simulink model "level1_challenge2a"  (R2023b)
settings: Solver=VariableStepAuto  StartTime=0.0  StopTime=600  RelTol=1e-3
settings Model: Creator=evreng  LastModifiedBy=evreng

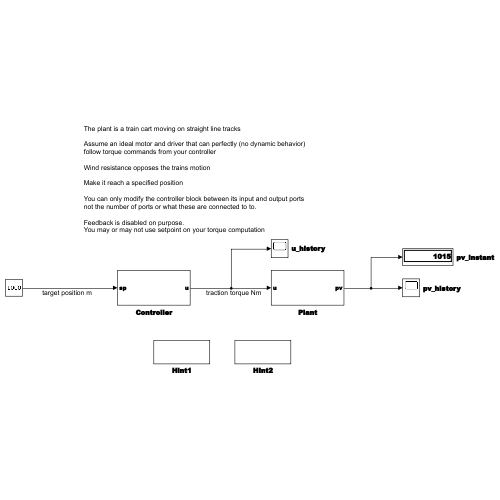
[thumbnail: Simulink's stored preview of the top-level diagram]
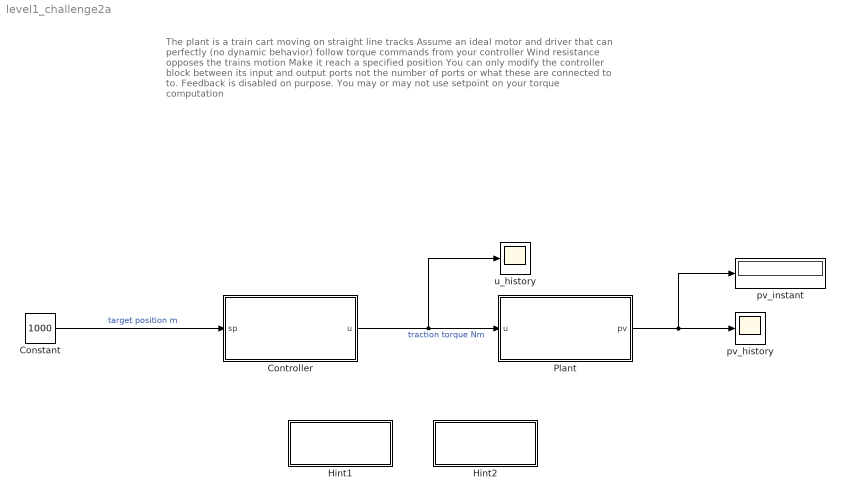
== system level1_challenge2a ==
  note: The plant is a train cart moving on straight line tracks
      |
      | Assume an ideal motor and driver that can perfectly (no dynamic behavior) follow torque commands from your controller
      |
      | Wind resistance opposes the trains motion
      |
      | Make it reach a specified position
      |
      | You can only modify the controller block between its input and output ports
      | not the number of ports or what these are connected to to.
      |
      | Feedback is disabled on purpose.
      | You may or may not use setpoint on your torque computation
  Constant : Constant  Value=1000
  Controller : Subsystem
  Hint1 : Subsystem
  Hint2 : Subsystem
  Plant : Subsystem
  pv_history : Scope
  pv_instant : Display
  u_history : Scope
  wires:
  Controller/1(u) -> Plant/1(u), u_history/1  "traction torque Nm"
  Constant/1 -> Controller/1(sp)  "target position m"
  Plant/1(pv) -> pv_history/1, pv_instant/1

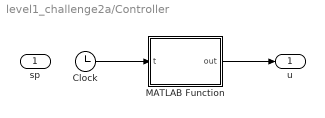
== system level1_challenge2a/Controller ==
  sp : Inport
  Clock : Clock
  MATLAB Function : MATLAB Function  TreatAsAtomicUnit=on
  u : Outport
  wires:
  MATLAB Function/1(out) -> u/1
  Clock/1 -> MATLAB Function/1(t)

== system level1_challenge2a/Hint1 ==
  note: A constant torque is no longer a solution. You need to decelarate and stop. Since air drag reduces as you slow down, you need to actively brake (or apply negative torque) at some point. Without feedback, the real problem is finding out when to and how hard to do so. Note that braking and negative torque are not the same thing. You will not go backwards when you brake. With negative torque, you will also need to remove the negative torque at some point.

== system level1_challenge2a/Hint2 ==
  note: You may want to use a predictor. That is, make your own model predicting poisition and take pseudo-feedback to reduce trial and error misery

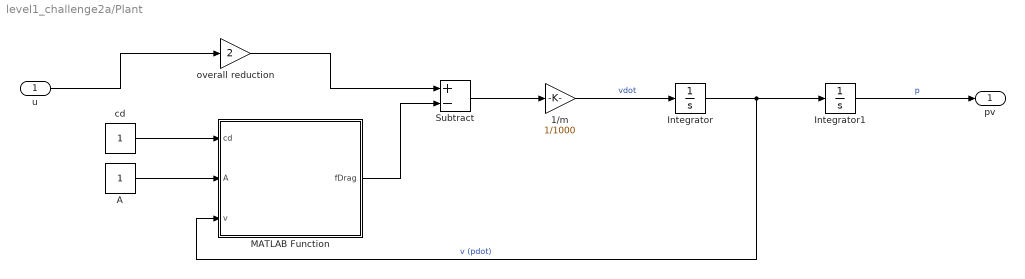
== system level1_challenge2a/Plant ==
  u : Inport
  1/m : Gain  Gain=1/1000
  A : Constant
  Integrator : Integrator
  Integrator1 : Integrator
  MATLAB Function : MATLAB Function  TreatAsAtomicUnit=on
  Subtract : Sum  Inputs=+-
  cd : Constant
  overall reduction : Gain  Gain=2
  pv : Outport
  wires:
  u/1 -> overall reduction/1
  1/m/1 -> Integrator/1  "vdot"
  Integrator/1 -> MATLAB Function/3(v), Integrator1/1  "v (pdot)"
  cd/1 -> MATLAB Function/1(cd)
  A/1 -> MATLAB Function/2(A)
  MATLAB Function/1(fDrag) -> Subtract/2
  Subtract/1 -> 1/m/1
  overall reduction/1 -> Subtract/1
  Integrator1/1 -> pv/1  "p"

== matlab function level1_challenge2a/Plant/MATLAB Function ==
  data: cd input; fDrag output; A input; v input
function fDrag = airDrag(cd, A, v)
fDrag = 0.5 * cd * A * v ^ 2 * sign(v);

== matlab function level1_challenge2a/Controller/MATLAB Function ==
  data: t input; out output
function out = fcn(t)
if t < 25
    out = 500;
elseif t < 100
    out = -124.5;
else
    out = 0;
end
